simulink library "GenericINSLibrary"  (R2020b)
settings: Solver=VariableStepAuto  StartTime=0.0  StopTime=10.0  RelTol=1e-3
libraries: simulink x44
(part 1 of 6)
settings Model: Creator=Scythe  LastModifiedBy=Scythe
settings DataIOCC: ReturnWorkspaceOutputs=off
settings DebuggingCC: ArithmeticOperatorsInVariantConditions=warning
settings SFSimCC: CustomCodeUndefinedFunction=UseInterfaceOnly

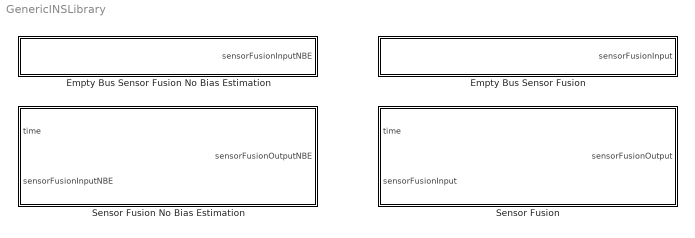
== system GenericINSLibrary ==
  Empty Bus Sensor Fusion : Subsystem
      mask help:
      | Create an empty bus to be used as input for the sensor fusion. By default all measurement values are set to zero and all standard deviations are set to one. A default sensor position is zero and a default sensor orientation equals to an identity matrix.<br><br>
      |
      | Assign values for all fields in the nested initialization bus and assign values for all fields in the nested sensor/IMU bus. All remaining nested sensor busses can optionally be assigned.<br><br>
      |
      | Note that a sensor measurement is only used, if the timestamp of the corresponding sensor increases.
      | Note that the initial state must be given with respect to the position of the IMU.
      mask DialogControl DescGroupVar Prompt: Empty Bus - Sensor Fusion Input
      mask Display: disp('Empty Bus\nSensor Fusion')
  Empty Bus Sensor Fusion No Bias Estimation : Subsystem
      mask help:
      | Create an empty bus to be used as input for the sensor fusion (no bias estimation). By default all measurement values are set to zero and all standard deviations are set to one. A default sensor position is zero and a default sensor orientation equals to an identity matrix.<br><br>
      |
      | Assign values for all fields in the nested initialization bus and assign values for all fields in the nested sensor/IMU bus. All remaining nested sensor busses can optionally be assigned.<br><br>
      |
      | Note that a sensor measurement is only used, if the timestamp of the corresponding sensor increases.
      | Note that the initial state must be given with respect to the position of the IMU.
      mask DialogControl DescGroupVar Prompt: Empty Bus - Sensor Fusion Input (No Bias Estimation)
      mask Display: disp('Empty Bus\nSensor Fusion\n(No Bias Estimation)')
  Sensor Fusion : Subsystem
      mask help:
      | The sensor fusion algorithm that uses multiple sensor data to estimate a motion state and also the inertial sensor biases. An IMU is strictly required to make predictions of the motion. If the IMU is not available for 200 milliseconds, then the filter enters an invalid state and has to be reset/re-initialized. The filter starts in an invalid state and has to be initialized by assigning values to the nested initialization bus and setting the reset flag to true. As long as the reset flag is set to true, the filter is initialized. The sensor fusion output is valid if the filter is initialized and least one prediction using IMU data has been performed.<br><br>
      |
      | <b>INPUT</b><br>
      | <b>time</b><br>
      | The input time source (in seconds) that is used to check for timeout. This time must be monotonically increasing.<br><br>
      |
      | <b>sensorFusionInput</b><br>
      | A bus representing the input to the sensor fusion. An empty input bus can be created by the <i>EmptyBusSensorFusionInput</i> block. Take a look to the mask of this block for more information.<br><br>
      |
      | <b>OUTPUT</b><br>
      | <b>sensorFusionOutput</b><br>
      | A bus representing the output of the sensor fusion. The nested state bus contains the state estimation. The nested info bus contains a valid flag that specifies whether the sensor fusion output is valid or not. Note that the filter gets invalid if IMU measurements timed out.
      mask DialogControl DescGroupVar Prompt: Sensor Fusion
      mask Display: disp('Generic INS\n\nSensor Fusion');
  Sensor Fusion No Bias Estimation : Subsystem
      mask help:
      | The sensor fusion algorithm that uses multiple sensor data to estimate a motion state. An IMU is strictly required to make predictions of the motion. If the IMU is not available for 200 milliseconds, then the filter enters an invalid state and has to be reset/re-initialized. The filter starts in an invalid state and has to be initialized by assigning values to the nested initialization bus and setting the reset flag to true. As long as the reset flag is set to true, the filter is initialized. The sensor fusion output is valid if the filter is initialized and least one prediction using IMU data has been performed.<br><br>
      |
      | <b>INPUT</b><br>
      | <b>time</b><br>
      | The input time source (in seconds) that is used to check for timeout. This time must be monotonically increasing.<br><br>
      |
      | <b>sensorFusionInputNBE</b><br>
      | A bus representing the input to the sensor fusion (no bias estimation). An empty input bus can be created by the <i>EmptyBusSensorFusionInput</i> block. Take a look to the mask of this block for more information.<br><br>
      |
      | <b>OUTPUT</b><br>
      | <b>sensorFusionOutputNBE</b><br>
      | A bus representing the output of the sensor fusion (no bias estimation). The nested state bus contains the state estimation. The nested info bus contains a valid flag that specifies whether the sensor fusion output is valid or not. Note that the filter gets invalid if IMU measurements timed out.
      mask DialogControl DescGroupVar Prompt: Sensor Fusion (No Bias Estimation)
      mask Display: disp('Generic INS\n\nSensor Fusion\n(No Bias Estimation)');

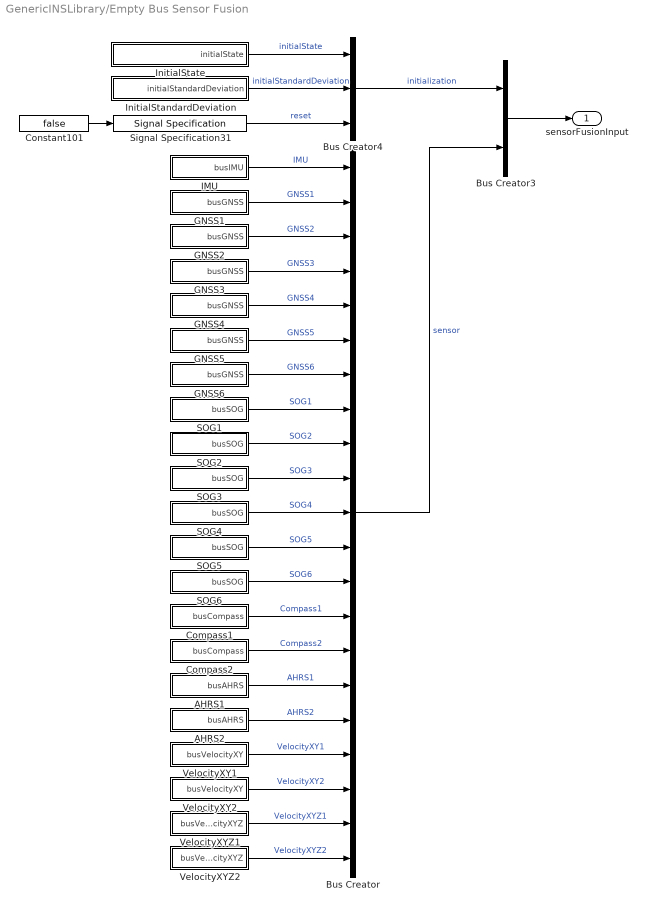
== system GenericINSLibrary/Empty Bus Sensor Fusion ==
  AHRS1 : Subsystem
  AHRS2 : Subsystem
  Bus Creator : BusCreator  Inputs=21
  Bus Creator3 : BusCreator  Inputs=2
  Bus Creator4 : BusCreator  Inputs=3
  Compass1 : Subsystem
  Compass2 : Subsystem
  Constant101 : Constant  Value=false  OutDataTypeStr=boolean
  GNSS1 : Subsystem
  GNSS2 : Subsystem
  GNSS3 : Subsystem
  GNSS4 : Subsystem
  GNSS5 : Subsystem
  GNSS6 : Subsystem
  IMU : Subsystem
  InitialStandardDeviation : Subsystem
  InitialState : Subsystem
  SOG1 : Subsystem
  SOG2 : Subsystem
  SOG3 : Subsystem
  SOG4 : Subsystem
  SOG5 : Subsystem
  SOG6 : Subsystem
  Signal Specification31 : SignalSpecification  OutDataTypeStr=boolean  Dimensions=1
  VelocityXY1 : Subsystem
  VelocityXY2 : Subsystem
  VelocityXYZ1 : Subsystem
  VelocityXYZ2 : Subsystem
  sensorFusionInput : Outport
  wires:
  Bus Creator3/1 -> sensorFusionInput/1
  SOG6/1(busSOG) -> Bus Creator/13  "SOG6"
  AHRS1/1(busAHRS) -> Bus Creator/16  "AHRS1"
  VelocityXY1/1(busVelocityXY) -> Bus Creator/18  "VelocityXY1"
  VelocityXYZ1/1(busVelocityXYZ) -> Bus Creator/20  "VelocityXYZ1"
  SOG5/1(busSOG) -> Bus Creator/12  "SOG5"
  VelocityXY2/1(busVelocityXY) -> Bus Creator/19  "VelocityXY2"
  GNSS4/1(busGNSS) -> Bus Creator/5  "GNSS4"
  GNSS2/1(busGNSS) -> Bus Creator/3  "GNSS2"
  GNSS6/1(busGNSS) -> Bus Creator/7  "GNSS6"
  InitialStandardDeviation/1(initialStandardDeviation) -> Bus Creator4/2  "initialStandardDeviation"
  Bus Creator/1 -> Bus Creator3/2  "sensor"
  SOG1/1(busSOG) -> Bus Creator/8  "SOG1"
  InitialState/1(initialState) -> Bus Creator4/1  "initialState"
  VelocityXYZ2/1(busVelocityXYZ) -> Bus Creator/21  "VelocityXYZ2"
  AHRS2/1(busAHRS) -> Bus Creator/17  "AHRS2"
  Compass2/1(busCompass) -> Bus Creator/15  "Compass2"
  SOG4/1(busSOG) -> Bus Creator/11  "SOG4"
  SOG3/1(busSOG) -> Bus Creator/10  "SOG3"
  Bus Creator4/1 -> Bus Creator3/1  "initialization"
  GNSS5/1(busGNSS) -> Bus Creator/6  "GNSS5"
  Constant101/1 -> Signal Specification31/1
  GNSS3/1(busGNSS) -> Bus Creator/4  "GNSS3"
  Compass1/1(busCompass) -> Bus Creator/14  "Compass1"
  GNSS1/1(busGNSS) -> Bus Creator/2  "GNSS1"
  Signal Specification31/1 -> Bus Creator4/3  "reset"
  IMU/1(busIMU) -> Bus Creator/1  "IMU"
  SOG2/1(busSOG) -> Bus Creator/9  "SOG2"

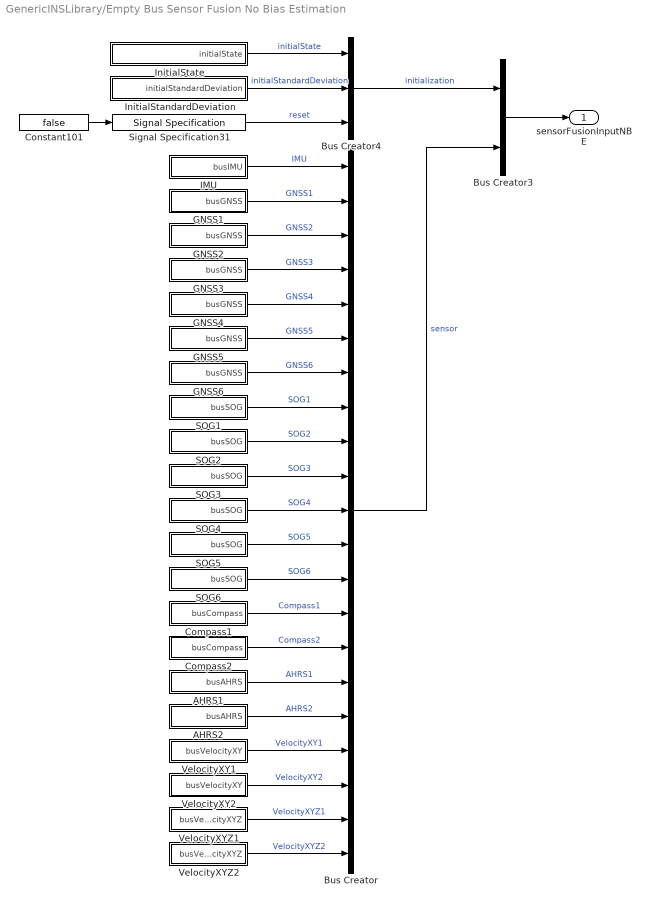
== system GenericINSLibrary/Empty Bus Sensor Fusion No Bias Estimation ==
  AHRS1 : Subsystem
  AHRS2 : Subsystem
  Bus Creator : BusCreator  Inputs=21
  Bus Creator3 : BusCreator  Inputs=2
  Bus Creator4 : BusCreator  Inputs=3
  Compass1 : Subsystem
  Compass2 : Subsystem
  Constant101 : Constant  Value=false  OutDataTypeStr=boolean
  GNSS1 : Subsystem
  GNSS2 : Subsystem
  GNSS3 : Subsystem
  GNSS4 : Subsystem
  GNSS5 : Subsystem
  GNSS6 : Subsystem
  IMU : Subsystem
  InitialStandardDeviation : Subsystem
  InitialState : Subsystem
  SOG1 : Subsystem
  SOG2 : Subsystem
  SOG3 : Subsystem
  SOG4 : Subsystem
  SOG5 : Subsystem
  SOG6 : Subsystem
  Signal Specification31 : SignalSpecification  OutDataTypeStr=boolean  Dimensions=1
  VelocityXY1 : Subsystem
  VelocityXY2 : Subsystem
  VelocityXYZ1 : Subsystem
  VelocityXYZ2 : Subsystem
  sensorFusionInputNBE : Outport
  wires:
  SOG2/1(busSOG) -> Bus Creator/9  "SOG2"
  IMU/1(busIMU) -> Bus Creator/1  "IMU"
  Signal Specification31/1 -> Bus Creator4/3  "reset"
  GNSS1/1(busGNSS) -> Bus Creator/2  "GNSS1"
  Compass1/1(busCompass) -> Bus Creator/14  "Compass1"
  GNSS3/1(busGNSS) -> Bus Creator/4  "GNSS3"
  Constant101/1 -> Signal Specification31/1
  GNSS5/1(busGNSS) -> Bus Creator/6  "GNSS5"
  Bus Creator4/1 -> Bus Creator3/1  "initialization"
  SOG3/1(busSOG) -> Bus Creator/10  "SOG3"
  SOG4/1(busSOG) -> Bus Creator/11  "SOG4"
  Compass2/1(busCompass) -> Bus Creator/15  "Compass2"
  AHRS2/1(busAHRS) -> Bus Creator/17  "AHRS2"
  VelocityXYZ2/1(busVelocityXYZ) -> Bus Creator/21  "VelocityXYZ2"
  InitialState/1(initialState) -> Bus Creator4/1  "initialState"
  SOG1/1(busSOG) -> Bus Creator/8  "SOG1"
  Bus Creator/1 -> Bus Creator3/2  "sensor"
  InitialStandardDeviation/1(initialStandardDeviation) -> Bus Creator4/2  "initialStandardDeviation"
  GNSS6/1(busGNSS) -> Bus Creator/7  "GNSS6"
  GNSS2/1(busGNSS) -> Bus Creator/3  "GNSS2"
  GNSS4/1(busGNSS) -> Bus Creator/5  "GNSS4"
  VelocityXY2/1(busVelocityXY) -> Bus Creator/19  "VelocityXY2"
  SOG5/1(busSOG) -> Bus Creator/12  "SOG5"
  VelocityXYZ1/1(busVelocityXYZ) -> Bus Creator/20  "VelocityXYZ1"
  VelocityXY1/1(busVelocityXY) -> Bus Creator/18  "VelocityXY1"
  AHRS1/1(busAHRS) -> Bus Creator/16  "AHRS1"
  SOG6/1(busSOG) -> Bus Creator/13  "SOG6"
  Bus Creator3/1 -> sensorFusionInputNBE/1

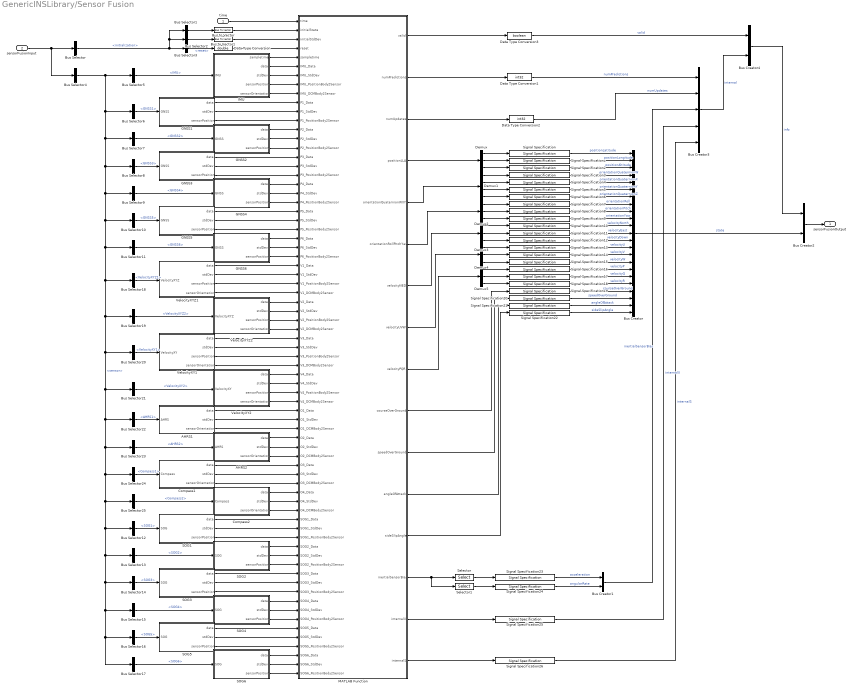
== system GenericINSLibrary/Sensor Fusion ==
  time : Inport  OutDataTypeStr=double  Unit=s  PortDimensions=1
  sensorFusionInput : Inport  Port=2
  AHRS1 : Subsystem
  AHRS2 : Subsystem
  Bus Creator : BusCreator  Inputs=23
  Bus Creator1 : BusCreator  Inputs=2
  Bus Creator2 : BusCreator  Inputs=2
  Bus Creator3 : BusCreator  Inputs=5
  Bus Creator4 : BusCreator  Inputs=2
  Bus Selector : BusSelector  OutputSignals=initialization
  Bus Selector1 : BusSelector  OutputSignals=initialState  OutputAsBus=on
  Bus Selector10 : BusSelector  OutputSignals=GNSS5
  Bus Selector11 : BusSelector  OutputSignals=GNSS6
  Bus Selector12 : BusSelector  OutputSignals=SOG1
  Bus Selector13 : BusSelector  OutputSignals=SOG2
  Bus Selector14 : BusSelector  OutputSignals=SOG3
  Bus Selector15 : BusSelector  OutputSignals=SOG4
  Bus Selector16 : BusSelector  OutputSignals=SOG5
  Bus Selector17 : BusSelector  OutputSignals=SOG6
  Bus Selector18 : BusSelector  OutputSignals=VelocityXYZ1
  Bus Selector19 : BusSelector  OutputSignals=VelocityXYZ2
  Bus Selector2 : BusSelector  OutputSignals=initialStandardDeviation  OutputAsBus=on
  Bus Selector20 : BusSelector  OutputSignals=VelocityXY1
  Bus Selector21 : BusSelector  OutputSignals=VelocityXY2
  Bus Selector22 : BusSelector  OutputSignals=AHRS1
  Bus Selector23 : BusSelector  OutputSignals=AHRS2
  Bus Selector24 : BusSelector  OutputSignals=Compass1
  Bus Selector25 : BusSelector  OutputSignals=Compass2
  Bus Selector3 : BusSelector  OutputSignals=reset
  Bus Selector4 : BusSelector  OutputSignals=sensor
  Bus Selector5 : BusSelector  OutputSignals=IMU
  Bus Selector6 : BusSelector  OutputSignals=GNSS1
  Bus Selector7 : BusSelector  OutputSignals=GNSS2
  Bus Selector8 : BusSelector  OutputSignals=GNSS3
  Bus Selector9 : BusSelector  OutputSignals=GNSS4
  Bus to Vector : BusToVector
  Bus to Vector1 : BusToVector
  Compass1 : Subsystem
  Compass2 : Subsystem
  Data Type Conversion : DataTypeConversion  OutDataTypeStr=double
  Data Type Conversion1 : DataTypeConversion  OutDataTypeStr=int32
  Data Type Conversion2 : DataTypeConversion  OutDataTypeStr=int32
  Data Type Conversion3 : DataTypeConversion  OutDataTypeStr=boolean
  Demux{,2..5} (5 alike) : Demux  Outputs=3
  Demux1 : Demux
  GNSS1 : Subsystem
  GNSS2 : Subsystem
  GNSS3 : Subsystem
  GNSS4 : Subsystem
  GNSS5 : Subsystem
  GNSS6 : Subsystem
  IMU : Subsystem
  MATLAB Function : MATLAB Function  TreatAsAtomicUnit=on
  SOG1 : Subsystem
  SOG2 : Subsystem
  SOG3 : Subsystem
  SOG4 : Subsystem
  SOG5 : Subsystem
  SOG6 : Subsystem
  Selector : Selector  InputPortWidth=6  IndexOptions=Index vector (dialog)  Indices=1:3  OutputSizes=1
  Selector1 : Selector  InputPortWidth=6  IndexOptions=Index vector (dialog)  Indices=4:6  OutputSizes=1
  Signal Specification{,1,7..9,19,21..22} (8 alike) : SignalSpecification  OutDataTypeStr=double  Unit=rad  Dimensions=1
  Signal Specification{10..15,20} (7 alike) : SignalSpecification  OutDataTypeStr=double  Unit=m/s  Dimensions=1
  Signal Specification16 : SignalSpecification  OutDataTypeStr=double  Unit=rad/s  Dimensions=1
  Signal Specification17 : SignalSpecification  OutDataTypeStr=double  Unit=rad/s  Dimensions=1
  Signal Specification18 : SignalSpecification  OutDataTypeStr=double  Unit=rad/s  Dimensions=1
  Signal Specification2 : SignalSpecification  OutDataTypeStr=double  Unit=m  Dimensions=1
  Signal Specification23 : SignalSpecification  OutDataTypeStr=double  Unit=m/s^2  Dimensions=[3 1]
  Signal Specification24 : SignalSpecification  OutDataTypeStr=double  Unit=rad/s  Dimensions=[3 1]
  Signal Specification25 : SignalSpecification  OutDataTypeStr=double  Dimensions=[16 1]
  Signal Specification26 : SignalSpecification  OutDataTypeStr=double  Dimensions=[15 15]
  Signal Specification{3..6} (4 alike) : SignalSpecification  OutDataTypeStr=double  Dimensions=1
  VelocityXY1 : Subsystem
  VelocityXY2 : Subsystem
  VelocityXYZ1 : Subsystem
  VelocityXYZ2 : Subsystem
  sensorFusionOutput : Outport
  wires:
  Bus Selector24/1 -> Compass1/1(Compass)  "<Compass1>"
  Bus Selector7/1 -> GNSS2/1(GNSS)  "<GNSS2>"
  Bus Selector17/1 -> SOG6/1(SOG)  "<SOG6>"
  AHRS1/2(stdDev) -> MATLAB Function/45(O1_StdDev)
  Compass2/3(sensorOrientation) -> MATLAB Function/55(O4_DCMBody2Sensor)
  MATLAB Function/11(speedOverGround) -> Signal Specification20/1
  Selector/1 -> Signal Specification23/1
  AHRS2/2(stdDev) -> MATLAB Function/48(O2_StdDev)
  SOG4/3(sensorPosition) -> MATLAB Function/67(SOG4_PositionBody2Sensor)
  Bus Selector20/1 -> VelocityXY1/1(VelocityXY)  "<VelocityXY1>"
  Demux/3 -> Signal Specification2/1
  Bus Selector16/1 -> SOG5/1(SOG)  "<SOG5>"
  Demux4/2 -> Signal Specification14/1
  SOG3/1(data) -> MATLAB Function/62(SOG3_Data)
  Bus Selector25/1 -> Compass2/1(Compass)  "<Compass2>"
  VelocityXY1/3(sensorPosition) -> MATLAB Function/38(V3_PositionBody2Sensor)
  VelocityXYZ2/2(stdDev) -> MATLAB Function/33(V2_StdDev)
  Signal Specification10/1 -> Bus Creator/11  "velocityNorth"
  GNSS2/1(data) -> MATLAB Function/13(P2_Data)
  Signal Specification3/1 -> Bus Creator/4  "orientationQuaternionW"
  AHRS1/1(data) -> MATLAB Function/44(O1_Data)
  Demux5/2 -> Signal Specification17/1
  SOG4/1(data) -> MATLAB Function/65(SOG4_Data)
  GNSS2/2(stdDev) -> MATLAB Function/14(P2_StdDev)
  Data Type Conversion3/1 -> Bus Creator4/1  "valid"
  MATLAB Function/6(orientationRollPitchYaw) -> Demux2/1
  Demux3/2 -> Signal Specification11/1
  AHRS2/1(data) -> MATLAB Function/47(O2_Data)
  GNSS6/2(stdDev) -> MATLAB Function/26(P6_StdDev)
  Compass1/2(stdDev) -> MATLAB Function/51(O3_StdDev)
  Demux1/2 -> Signal Specification4/1
  Signal Specification22/1 -> Bus Creator/23  "sideSlipAngle"
  Bus Selector1/1 -> Bus to Vector/1
  Bus Selector18/1 -> VelocityXYZ1/1(VelocityXYZ)  "<VelocityXYZ1>"
  MATLAB Function/14(inertialSensorBias) -> Selector/1, Selector1/1
  GNSS6/1(data) -> MATLAB Function/25(P6_Data)
  Signal Specification11/1 -> Bus Creator/12  "velocityEast"
  GNSS1/3(sensorPosition) -> MATLAB Function/12(P1_PositionBody2Sensor)
  Compass1/1(data) -> MATLAB Function/50(O3_Data)
  Compass2/2(stdDev) -> MATLAB Function/54(O4_StdDev)
  Demux1/4 -> Signal Specification6/1
  Demux2/3 -> Signal Specification9/1
  Demux1/3 -> Signal Specification5/1
  Bus Selector13/1 -> SOG2/1(SOG)  "<SOG2>"
  Bus Selector9/1 -> GNSS4/1(GNSS)  "<GNSS4>"
  Data Type Conversion2/1 -> Bus Creator3/2  "numUpdates"
  Bus Creator2/1 -> sensorFusionOutput/1
  Bus to Vector/1 -> MATLAB Function/2(initialState)
  VelocityXYZ1/1(data) -> MATLAB Function/28(V1_Data)
  Signal Specification18/1 -> Bus Creator/19  "velocityR"
  SOG2/3(sensorPosition) -> MATLAB Function/61(SOG2_PositionBody2Sensor)
  SOG6/2(stdDev) -> MATLAB Function/72(SOG6_StdDev)
  SOG3/3(sensorPosition) -> MATLAB Function/64(SOG3_PositionBody2Sensor)
  Signal Specification7/1 -> Bus Creator/8  "orientationRoll"
  Bus to Vector1/1 -> MATLAB Function/3(initialStdDev)
  Bus Creator4/1 -> Bus Creator2/1  "info"
  Signal Specification6/1 -> Bus Creator/7  "orientationQuaternionZ"
  MATLAB Function/4(positionLLA) -> Demux/1
  Bus Selector3/1 -> Data Type Conversion/1  "<reset>"
  GNSS4/3(sensorPosition) -> MATLAB Function/21(P4_PositionBody2Sensor)
  Bus Selector11/1 -> GNSS6/1(GNSS)  "<GNSS6>"
  Signal Specification25/1 -> Bus Creator3/4  "internalX"
  Demux5/1 -> Signal Specification16/1
  Compass2/1(data) -> MATLAB Function/53(O4_Data)
  Bus Creator3/1 -> Bus Creator4/2  "internal"
  Signal Specification17/1 -> Bus Creator/18  "velocityQ"
  time/1 -> MATLAB Function/1(time)
  Demux4/3 -> Signal Specification15/1
  MATLAB Function/13(sideSlipAngle) -> Signal Specification22/1
  MATLAB Function/9(velocityPQR) -> Demux5/1
  Bus Selector/1 -> Bus Selector3/1, Bus Selector1/1, Bus Selector2/1  "<initialization>"
  VelocityXYZ1/2(stdDev) -> MATLAB Function/29(V1_StdDev)
  MATLAB Function/16(internalS) -> Signal Specification26/1
  Demux/1 -> Signal Specification/1
  GNSS5/2(stdDev) -> MATLAB Function/23(P5_StdDev)
  Signal Specification15/1 -> Bus Creator/16  "velocityW"
  SOG5/3(sensorPosition) -> MATLAB Function/70(SOG5_PositionBody2Sensor)
  MATLAB Function/5(orientationQuaternionWXYZ) -> Demux1/1
  GNSS2/3(sensorPosition) -> MATLAB Function/15(P2_PositionBody2Sensor)
  Bus Creator/1 -> Bus Creator2/2  "state"
  MATLAB Function/10(courseOverGround) -> Signal Specification19/1
  VelocityXY1/1(data) -> MATLAB Function/36(V3_Data)
  GNSS4/1(data) -> MATLAB Function/19(P4_Data)
  Demux3/3 -> Signal Specification12/1
  SOG5/1(data) -> MATLAB Function/68(SOG5_Data)
  Signal Specification21/1 -> Bus Creator/22  "angleOfAttack"
  Bus Selector12/1 -> SOG1/1(SOG)  "<SOG1>"
  Demux2/1 -> Signal Specification7/1
  IMU/3(stdDev) -> MATLAB Function/7(IMU_StdDev)
  Demux/2 -> Signal Specification1/1
  SOG2/2(stdDev) -> MATLAB Function/60(SOG2_StdDev)
  Bus Selector8/1 -> GNSS3/1(GNSS)  "<GNSS3>"
  VelocityXY1/4(sensorOrientation) -> MATLAB Function/39(V3_DCMBody2Sensor)
  Signal Specification16/1 -> Bus Creator/17  "velocityP"
  GNSS1/2(stdDev) -> MATLAB Function/11(P1_StdDev)
  SOG1/1(data) -> MATLAB Function/56(SOG1_Data)
  SOG5/2(stdDev) -> MATLAB Function/69(SOG5_StdDev)
  Data Type Conversion1/1 -> Bus Creator3/1  "numPredictions"
  Bus Selector6/1 -> GNSS1/1(GNSS)  "<GNSS1>"
  GNSS6/3(sensorPosition) -> MATLAB Function/27(P6_PositionBody2Sensor)
  sensorFusionInput/1 -> Bus Selector/1, Bus Selector4/1
  MATLAB Function/1(valid) -> Data Type Conversion3/1
  Signal Specification1/1 -> Bus Creator/2  "positionLongitude"
  SOG6/3(sensorPosition) -> MATLAB Function/73(SOG6_PositionBody2Sensor)
  VelocityXY2/3(sensorPosition) -> MATLAB Function/42(V4_PositionBody2Sensor)
  IMU/1(sampletime) -> MATLAB Function/5(sampletime)
  MATLAB Function/15(internalX) -> Signal Specification25/1
  Signal Specification8/1 -> Bus Creator/9  "orientationPitch"
  Bus Selector4/1 -> Bus Selector5/1, Bus Selector6/1, Bus Selector7/1, Bus Selector8/1, Bus Selector9/1, Bus Selector10/1, Bus Selector11/1, Bus Selector18/1, Bus Selector19/1, Bus Selector22/1, Bus Selector12/1, Bus Selector13/1, Bus Selector17/1, Bus Selector16/1, Bus Selector15/1, Bus Selector14/1, Bus Selector25/1, Bus Selector24/1, Bus Selector23/1, Bus Selector21/1, Bus Selector20/1  "<sensor>"
  GNSS4/2(stdDev) -> MATLAB Function/20(P4_StdDev)
  Bus Selector15/1 -> SOG4/1(SOG)  "<SOG4>"
  Demux3/1 -> Signal Specification10/1
  Signal Specification26/1 -> Bus Creator3/5  "internalS"
  Signal Specification9/1 -> Bus Creator/10  "orientationYaw"
  Bus Selector5/1 -> IMU/1(IMU)  "<IMU>"
  Data Type Conversion/1 -> MATLAB Function/4(reset)
  Signal Specification4/1 -> Bus Creator/5  "orientationQuaternionX"
  SOG4/2(stdDev) -> MATLAB Function/66(SOG4_StdDev)
  Bus Selector2/1 -> Bus to Vector1/1
  Compass1/3(sensorOrientation) -> MATLAB Function/52(O3_DCMBody2Sensor)
  GNSS5/3(sensorPosition) -> MATLAB Function/24(P5_PositionBody2Sensor)
  VelocityXY2/4(sensorOrientation) -> MATLAB Function/43(V4_DCMBody2Sensor)
  SOG6/1(data) -> MATLAB Function/71(SOG6_Data)
  Demux5/3 -> Signal Specification18/1
  Bus Selector10/1 -> GNSS5/1(GNSS)  "<GNSS5>"
  Signal Specification12/1 -> Bus Creator/13  "velocityDown"
  VelocityXYZ1/4(sensorOrientation) -> MATLAB Function/31(V1_DCMBody2Sensor)
  IMU/5(sensorOrientation) -> MATLAB Function/9(IMU_DCMBody2Sensor)
  Signal Specification20/1 -> Bus Creator/21  "speedOverGround"
  SOG1/3(sensorPosition) -> MATLAB Function/58(SOG1_PositionBody2Sensor)
  SOG3/2(stdDev) -> MATLAB Function/63(SOG3_StdDev)
  Signal Specification/1 -> Bus Creator/1  "positionLatitude"
  IMU/2(data) -> MATLAB Function/6(IMU_Data)
  Demux4/1 -> Signal Specification13/1
  Signal Specification14/1 -> Bus Creator/15  "velocityV"
  VelocityXY2/2(stdDev) -> MATLAB Function/41(V4_StdDev)
  GNSS1/1(data) -> MATLAB Function/10(P1_Data)
  Bus Creator1/1 -> Bus Creator3/3  "inertialSensorBias"
  GNSS3/3(sensorPosition) -> MATLAB Function/18(P3_PositionBody2Sensor)
  GNSS3/1(data) -> MATLAB Function/16(P3_Data)
  Demux1/1 -> Signal Specification3/1
  VelocityXYZ2/4(sensorOrientation) -> MATLAB Function/35(V2_DCMBody2Sensor)
  VelocityXYZ2/3(sensorPosition) -> MATLAB Function/34(V2_PositionBody2Sensor)
  Signal Specification24/1 -> Bus Creator1/2  "angularRate"
  VelocityXYZ2/1(data) -> MATLAB Function/32(V2_Data)
  MATLAB Function/3(numUpdates) -> Data Type Conversion2/1
  VelocityXY1/2(stdDev) -> MATLAB Function/37(V3_StdDev)
  GNSS3/2(stdDev) -> MATLAB Function/17(P3_StdDev)
  Signal Specification13/1 -> Bus Creator/14  "velocityU"
  Signal Specification19/1 -> Bus Creator/20  "courseOverGround"
  Signal Specification2/1 -> Bus Creator/3  "positionAltitude"
  SOG1/2(stdDev) -> MATLAB Function/57(SOG1_StdDev)
  IMU/4(sensorPosition) -> MATLAB Function/8(IMU_PositionBody2Sensor)
  Bus Selector19/1 -> VelocityXYZ2/1(VelocityXYZ)  "<VelocityXYZ2>"
  MATLAB Function/7(velocityNED) -> Demux3/1
  Bus Selector14/1 -> SOG3/1(SOG)  "<SOG3>"
  VelocityXYZ1/3(sensorPosition) -> MATLAB Function/30(V1_PositionBody2Sensor)
  AHRS1/3(sensorOrientation) -> MATLAB Function/46(O1_DCMBody2Sensor)
  GNSS5/1(data) -> MATLAB Function/22(P5_Data)
  SOG2/1(data) -> MATLAB Function/59(SOG2_Data)
  MATLAB Function/2(numPredictions) -> Data Type Conversion1/1
  AHRS2/3(sensorOrientation) -> MATLAB Function/49(O2_DCMBody2Sensor)
  Selector1/1 -> Signal Specification24/1
  MATLAB Function/8(velocityUVW) -> Demux4/1
  Bus Selector22/1 -> AHRS1/1(AHRS)  "<AHRS1>"
  Demux2/2 -> Signal Specification8/1
  MATLAB Function/12(angleOfAttack) -> Signal Specification21/1
  Signal Specification23/1 -> Bus Creator1/1  "acceleration"
  Bus Selector21/1 -> VelocityXY2/1(VelocityXY)  "<VelocityXY2>"
  Signal Specification5/1 -> Bus Creator/6  "orientationQuaternionY"
  VelocityXY2/1(data) -> MATLAB Function/40(V4_Data)
  Bus Selector23/1 -> AHRS2/1(AHRS)  "<AHRS2>"

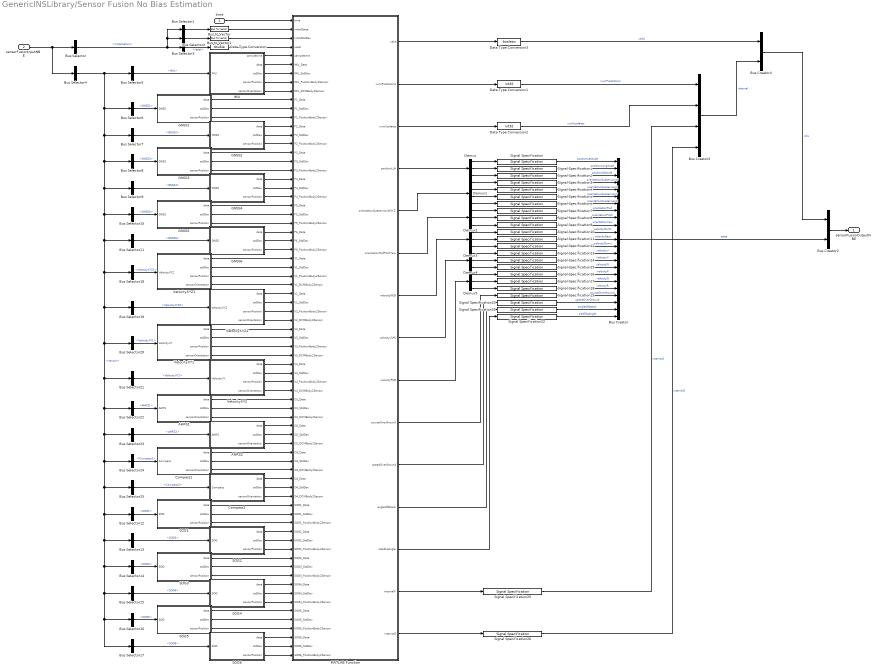
== system GenericINSLibrary/Sensor Fusion No Bias Estimation ==
  time : Inport  OutDataTypeStr=double  Unit=s  PortDimensions=1
  sensorFusionInputNBE : Inport  Port=2
  AHRS1 : Subsystem
  AHRS2 : Subsystem
  Bus Creator : BusCreator  Inputs=23
  Bus Creator2 : BusCreator  Inputs=2
  Bus Creator3 : BusCreator  Inputs=4
  Bus Creator4 : BusCreator  Inputs=2
  Bus Selector : BusSelector  OutputSignals=initialization
  Bus Selector1 : BusSelector  OutputSignals=initialState  OutputAsBus=on
  Bus Selector10 : BusSelector  OutputSignals=GNSS5
  Bus Selector11 : BusSelector  OutputSignals=GNSS6
  Bus Selector12 : BusSelector  OutputSignals=SOG1
  Bus Selector13 : BusSelector  OutputSignals=SOG2
  Bus Selector14 : BusSelector  OutputSignals=SOG3
  Bus Selector15 : BusSelector  OutputSignals=SOG4
  Bus Selector16 : BusSelector  OutputSignals=SOG5
  Bus Selector17 : BusSelector  OutputSignals=SOG6
  Bus Selector18 : BusSelector  OutputSignals=VelocityXYZ1
  Bus Selector19 : BusSelector  OutputSignals=VelocityXYZ2
  Bus Selector2 : BusSelector  OutputSignals=initialStandardDeviation  OutputAsBus=on
  Bus Selector20 : BusSelector  OutputSignals=VelocityXY1
  Bus Selector21 : BusSelector  OutputSignals=VelocityXY2
  Bus Selector22 : BusSelector  OutputSignals=AHRS1
  Bus Selector23 : BusSelector  OutputSignals=AHRS2
  Bus Selector24 : BusSelector  OutputSignals=Compass1
  Bus Selector25 : BusSelector  OutputSignals=Compass2
  Bus Selector3 : BusSelector  OutputSignals=reset
  Bus Selector4 : BusSelector  OutputSignals=sensor
  Bus Selector5 : BusSelector  OutputSignals=IMU
  Bus Selector6 : BusSelector  OutputSignals=GNSS1
  Bus Selector7 : BusSelector  OutputSignals=GNSS2
  Bus Selector8 : BusSelector  OutputSignals=GNSS3
  Bus Selector9 : BusSelector  OutputSignals=GNSS4
  Bus to Vector : BusToVector
  Bus to Vector1 : BusToVector
  Compass1 : Subsystem
  Compass2 : Subsystem
  Data Type Conversion : DataTypeConversion  OutDataTypeStr=double
  Data Type Conversion1 : DataTypeConversion  OutDataTypeStr=int32
  Data Type Conversion2 : DataTypeConversion  OutDataTypeStr=int32
  Data Type Conversion3 : DataTypeConversion  OutDataTypeStr=boolean
  Demux{,2..5} (5 alike) : Demux  Outputs=3
  Demux1 : Demux
  GNSS1 : Subsystem
  GNSS2 : Subsystem
  GNSS3 : Subsystem
  GNSS4 : Subsystem
  GNSS5 : Subsystem
  GNSS6 : Subsystem
  IMU : Subsystem
  MATLAB Function : MATLAB Function  TreatAsAtomicUnit=on
  SOG1 : Subsystem
  SOG2 : Subsystem
  SOG3 : Subsystem
  SOG4 : Subsystem
  SOG5 : Subsystem
  SOG6 : Subsystem
  Signal Specification{,1,7..9,19,21..22} (8 alike) : SignalSpecification  OutDataTypeStr=double  Unit=rad  Dimensions=1
  Signal Specification{10..15,20} (7 alike) : SignalSpecification  OutDataTypeStr=double  Unit=m/s  Dimensions=1
  Signal Specification16 : SignalSpecification  OutDataTypeStr=double  Unit=rad/s  Dimensions=1
  Signal Specification17 : SignalSpecification  OutDataTypeStr=double  Unit=rad/s  Dimensions=1
  Signal Specification18 : SignalSpecification  OutDataTypeStr=double  Unit=rad/s  Dimensions=1
  Signal Specification2 : SignalSpecification  OutDataTypeStr=double  Unit=m  Dimensions=1
  Signal Specification25 : SignalSpecification  OutDataTypeStr=double  Dimensions=[10 1]
  Signal Specification26 : SignalSpecification  OutDataTypeStr=double  Dimensions=[9 9]
  Signal Specification{3..6} (4 alike) : SignalSpecification  OutDataTypeStr=double  Dimensions=1
  VelocityXY1 : Subsystem
  VelocityXY2 : Subsystem
  VelocityXYZ1 : Subsystem
  VelocityXYZ2 : Subsystem
  sensorFusionOutputNBE : Outport
  wires:
  Bus Selector23/1 -> AHRS2/1(AHRS)  "<AHRS2>"
  VelocityXY2/1(data) -> MATLAB Function/40(V4_Data)
  Signal Specification5/1 -> Bus Creator/6  "orientationQuaternionY"
  Bus Selector21/1 -> VelocityXY2/1(VelocityXY)  "<VelocityXY2>"
  MATLAB Function/12(angleOfAttack) -> Signal Specification21/1
  Demux2/2 -> Signal Specification8/1
  Bus Selector22/1 -> AHRS1/1(AHRS)  "<AHRS1>"
  MATLAB Function/8(velocityUVW) -> Demux4/1
  AHRS2/3(sensorOrientation) -> MATLAB Function/49(O2_DCMBody2Sensor)
  MATLAB Function/2(numPredictions) -> Data Type Conversion1/1
  SOG2/1(data) -> MATLAB Function/59(SOG2_Data)
  GNSS5/1(data) -> MATLAB Function/22(P5_Data)
  AHRS1/3(sensorOrientation) -> MATLAB Function/46(O1_DCMBody2Sensor)
  VelocityXYZ1/3(sensorPosition) -> MATLAB Function/30(V1_PositionBody2Sensor)
  Bus Selector14/1 -> SOG3/1(SOG)  "<SOG3>"
  MATLAB Function/7(velocityNED) -> Demux3/1
  Bus Selector19/1 -> VelocityXYZ2/1(VelocityXYZ)  "<VelocityXYZ2>"
  IMU/4(sensorPosition) -> MATLAB Function/8(IMU_PositionBody2Sensor)
  SOG1/2(stdDev) -> MATLAB Function/57(SOG1_StdDev)
  Signal Specification2/1 -> Bus Creator/3  "positionAltitude"
  Signal Specification19/1 -> Bus Creator/20  "courseOverGround"
  Signal Specification13/1 -> Bus Creator/14  "velocityU"
  GNSS3/2(stdDev) -> MATLAB Function/17(P3_StdDev)
  VelocityXY1/2(stdDev) -> MATLAB Function/37(V3_StdDev)
  MATLAB Function/3(numUpdates) -> Data Type Conversion2/1
  VelocityXYZ2/1(data) -> MATLAB Function/32(V2_Data)
  VelocityXYZ2/3(sensorPosition) -> MATLAB Function/34(V2_PositionBody2Sensor)
  VelocityXYZ2/4(sensorOrientation) -> MATLAB Function/35(V2_DCMBody2Sensor)
  Demux1/1 -> Signal Specification3/1
  GNSS3/1(data) -> MATLAB Function/16(P3_Data)
  GNSS3/3(sensorPosition) -> MATLAB Function/18(P3_PositionBody2Sensor)
  GNSS1/1(data) -> MATLAB Function/10(P1_Data)
  VelocityXY2/2(stdDev) -> MATLAB Function/41(V4_StdDev)
  Signal Specification14/1 -> Bus Creator/15  "velocityV"
  Demux4/1 -> Signal Specification13/1
  IMU/2(data) -> MATLAB Function/6(IMU_Data)
  Signal Specification/1 -> Bus Creator/1  "positionLatitude"
  SOG3/2(stdDev) -> MATLAB Function/63(SOG3_StdDev)
  SOG1/3(sensorPosition) -> MATLAB Function/58(SOG1_PositionBody2Sensor)
  Signal Specification20/1 -> Bus Creator/21  "speedOverGround"
  IMU/5(sensorOrientation) -> MATLAB Function/9(IMU_DCMBody2Sensor)
  VelocityXYZ1/4(sensorOrientation) -> MATLAB Function/31(V1_DCMBody2Sensor)
  Signal Specification12/1 -> Bus Creator/13  "velocityDown"
  Bus Selector10/1 -> GNSS5/1(GNSS)  "<GNSS5>"
  Demux5/3 -> Signal Specification18/1
  SOG6/1(data) -> MATLAB Function/71(SOG6_Data)
  VelocityXY2/4(sensorOrientation) -> MATLAB Function/43(V4_DCMBody2Sensor)
  GNSS5/3(sensorPosition) -> MATLAB Function/24(P5_PositionBody2Sensor)
  Compass1/3(sensorOrientation) -> MATLAB Function/52(O3_DCMBody2Sensor)
  Bus Selector2/1 -> Bus to Vector1/1
  SOG4/2(stdDev) -> MATLAB Function/66(SOG4_StdDev)
  Signal Specification4/1 -> Bus Creator/5  "orientationQuaternionX"
  Data Type Conversion/1 -> MATLAB Function/4(reset)
  Bus Selector5/1 -> IMU/1(IMU)  "<IMU>"
  Signal Specification9/1 -> Bus Creator/10  "orientationYaw"
  Signal Specification26/1 -> Bus Creator3/4  "internalS"
  Demux3/1 -> Signal Specification10/1
  Bus Selector15/1 -> SOG4/1(SOG)  "<SOG4>"
  GNSS4/2(stdDev) -> MATLAB Function/20(P4_StdDev)
  Bus Selector4/1 -> Bus Selector20/1, Bus Selector21/1, Bus Selector23/1, Bus Selector24/1, Bus Selector25/1, Bus Selector14/1, Bus Selector15/1, Bus Selector16/1, Bus Selector17/1, Bus Selector13/1, Bus Selector12/1, Bus Selector22/1, Bus Selector19/1, Bus Selector18/1, Bus Selector11/1, Bus Selector10/1, Bus Selector9/1, Bus Selector8/1, Bus Selector7/1, Bus Selector6/1, Bus Selector5/1  "<sensor>"
  Signal Specification8/1 -> Bus Creator/9  "orientationPitch"
  MATLAB Function/14(internalX) -> Signal Specification25/1
  IMU/1(sampletime) -> MATLAB Function/5(sampletime)
  VelocityXY2/3(sensorPosition) -> MATLAB Function/42(V4_PositionBody2Sensor)
  SOG6/3(sensorPosition) -> MATLAB Function/73(SOG6_PositionBody2Sensor)
  Signal Specification1/1 -> Bus Creator/2  "positionLongitude"
  MATLAB Function/1(valid) -> Data Type Conversion3/1
  sensorFusionInputNBE/1 -> Bus Selector4/1, Bus Selector/1
  GNSS6/3(sensorPosition) -> MATLAB Function/27(P6_PositionBody2Sensor)
  Bus Selector6/1 -> GNSS1/1(GNSS)  "<GNSS1>"
  Data Type Conversion1/1 -> Bus Creator3/1  "numPredictions"
  SOG5/2(stdDev) -> MATLAB Function/69(SOG5_StdDev)
  SOG1/1(data) -> MATLAB Function/56(SOG1_Data)
  GNSS1/2(stdDev) -> MATLAB Function/11(P1_StdDev)
  Signal Specification16/1 -> Bus Creator/17  "velocityP"
  VelocityXY1/4(sensorOrientation) -> MATLAB Function/39(V3_DCMBody2Sensor)
  Bus Selector8/1 -> GNSS3/1(GNSS)  "<GNSS3>"
  SOG2/2(stdDev) -> MATLAB Function/60(SOG2_StdDev)
  Demux/2 -> Signal Specification1/1
  IMU/3(stdDev) -> MATLAB Function/7(IMU_StdDev)
  Demux2/1 -> Signal Specification7/1
  Bus Selector12/1 -> SOG1/1(SOG)  "<SOG1>"
  Signal Specification21/1 -> Bus Creator/22  "angleOfAttack"
  SOG5/1(data) -> MATLAB Function/68(SOG5_Data)
  Demux3/3 -> Signal Specification12/1
  GNSS4/1(data) -> MATLAB Function/19(P4_Data)
  VelocityXY1/1(data) -> MATLAB Function/36(V3_Data)
  MATLAB Function/10(courseOverGround) -> Signal Specification19/1
  Bus Creator/1 -> Bus Creator2/2  "state"
  GNSS2/3(sensorPosition) -> MATLAB Function/15(P2_PositionBody2Sensor)
  MATLAB Function/5(orientationQuaternionWXYZ) -> Demux1/1
  SOG5/3(sensorPosition) -> MATLAB Function/70(SOG5_PositionBody2Sensor)
  Signal Specification15/1 -> Bus Creator/16  "velocityW"
  GNSS5/2(stdDev) -> MATLAB Function/23(P5_StdDev)
  Demux/1 -> Signal Specification/1
  MATLAB Function/15(internalS) -> Signal Specification26/1
  VelocityXYZ1/2(stdDev) -> MATLAB Function/29(V1_StdDev)
  Bus Selector/1 -> Bus Selector2/1, Bus Selector1/1, Bus Selector3/1  "<initialization>"
  MATLAB Function/9(velocityPQR) -> Demux5/1
  MATLAB Function/13(sideSlipAngle) -> Signal Specification22/1
  Demux4/3 -> Signal Specification15/1
  time/1 -> MATLAB Function/1(time)
  Signal Specification17/1 -> Bus Creator/18  "velocityQ"
  Bus Creator3/1 -> Bus Creator4/2  "internal"
  Compass2/1(data) -> MATLAB Function/53(O4_Data)
  Demux5/1 -> Signal Specification16/1
  Signal Specification25/1 -> Bus Creator3/3  "internalX"
  Bus Selector11/1 -> GNSS6/1(GNSS)  "<GNSS6>"
  GNSS4/3(sensorPosition) -> MATLAB Function/21(P4_PositionBody2Sensor)
  Bus Selector3/1 -> Data Type Conversion/1  "<reset>"
  MATLAB Function/4(positionLLA) -> Demux/1
  Signal Specification6/1 -> Bus Creator/7  "orientationQuaternionZ"
  Bus Creator4/1 -> Bus Creator2/1  "info"
  Bus to Vector1/1 -> MATLAB Function/3(initialStdDev)
  Signal Specification7/1 -> Bus Creator/8  "orientationRoll"
  SOG3/3(sensorPosition) -> MATLAB Function/64(SOG3_PositionBody2Sensor)
  SOG6/2(stdDev) -> MATLAB Function/72(SOG6_StdDev)
  SOG2/3(sensorPosition) -> MATLAB Function/61(SOG2_PositionBody2Sensor)
  Signal Specification18/1 -> Bus Creator/19  "velocityR"
  VelocityXYZ1/1(data) -> MATLAB Function/28(V1_Data)
  Bus to Vector/1 -> MATLAB Function/2(initialState)
  Bus Creator2/1 -> sensorFusionOutputNBE/1
  Data Type Conversion2/1 -> Bus Creator3/2  "numUpdates"
  Bus Selector9/1 -> GNSS4/1(GNSS)  "<GNSS4>"
  Bus Selector13/1 -> SOG2/1(SOG)  "<SOG2>"
  Demux1/3 -> Signal Specification5/1
  Demux2/3 -> Signal Specification9/1
  Demux1/4 -> Signal Specification6/1
  Compass2/2(stdDev) -> MATLAB Function/54(O4_StdDev)
  Compass1/1(data) -> MATLAB Function/50(O3_Data)
  GNSS1/3(sensorPosition) -> MATLAB Function/12(P1_PositionBody2Sensor)
  Signal Specification11/1 -> Bus Creator/12  "velocityEast"
  GNSS6/1(data) -> MATLAB Function/25(P6_Data)
  Bus Selector18/1 -> VelocityXYZ1/1(VelocityXYZ)  "<VelocityXYZ1>"
  Bus Selector1/1 -> Bus to Vector/1
  Signal Specification22/1 -> Bus Creator/23  "sideSlipAngle"
  Demux1/2 -> Signal Specification4/1
  Compass1/2(stdDev) -> MATLAB Function/51(O3_StdDev)
  GNSS6/2(stdDev) -> MATLAB Function/26(P6_StdDev)
  AHRS2/1(data) -> MATLAB Function/47(O2_Data)
  Demux3/2 -> Signal Specification11/1
  MATLAB Function/6(orientationRollPitchYaw) -> Demux2/1
  Data Type Conversion3/1 -> Bus Creator4/1  "valid"
  GNSS2/2(stdDev) -> MATLAB Function/14(P2_StdDev)
  SOG4/1(data) -> MATLAB Function/65(SOG4_Data)
  Demux5/2 -> Signal Specification17/1
  AHRS1/1(data) -> MATLAB Function/44(O1_Data)
  Signal Specification3/1 -> Bus Creator/4  "orientationQuaternionW"
  GNSS2/1(data) -> MATLAB Function/13(P2_Data)
  Signal Specification10/1 -> Bus Creator/11  "velocityNorth"
  VelocityXYZ2/2(stdDev) -> MATLAB Function/33(V2_StdDev)
  VelocityXY1/3(sensorPosition) -> MATLAB Function/38(V3_PositionBody2Sensor)
  Bus Selector25/1 -> Compass2/1(Compass)  "<Compass2>"
  SOG3/1(data) -> MATLAB Function/62(SOG3_Data)
  Demux4/2 -> Signal Specification14/1
  Bus Selector16/1 -> SOG5/1(SOG)  "<SOG5>"
  Demux/3 -> Signal Specification2/1
  Bus Selector20/1 -> VelocityXY1/1(VelocityXY)  "<VelocityXY1>"
  SOG4/3(sensorPosition) -> MATLAB Function/67(SOG4_PositionBody2Sensor)
  AHRS2/2(stdDev) -> MATLAB Function/48(O2_StdDev)
  MATLAB Function/11(speedOverGround) -> Signal Specification20/1
  Compass2/3(sensorOrientation) -> MATLAB Function/55(O4_DCMBody2Sensor)
  AHRS1/2(stdDev) -> MATLAB Function/45(O1_StdDev)
  Bus Selector17/1 -> SOG6/1(SOG)  "<SOG6>"
  Bus Selector7/1 -> GNSS2/1(GNSS)  "<GNSS2>"
  Bus Selector24/1 -> Compass1/1(Compass)  "<Compass1>"

== system GenericINSLibrary/Empty Bus Sensor Fusion/AHRS1 ==
  Bus Creator : BusCreator  Inputs=1
  Bus Creator1 : BusCreator  Inputs=3
  Bus Creator2 : BusCreator  Inputs=3
  Bus Creator3 : BusCreator  Inputs=4
  Constant1 : Constant  OutDataTypeStr=double
  Constant2 : Constant  OutDataTypeStr=double
  Constant{3..4,75..76} (4 alike) : Constant  Value=0  OutDataTypeStr=double
  Constant71 : Constant  Value=eye(3)  OutDataTypeStr=double
  Constant72 : Constant  OutDataTypeStr=double
  Signal Specification : SignalSpecification  OutDataTypeStr=double  Dimensions=[3 3]
  Signal Specification{1..3,5..7} (6 alike) : SignalSpecification  OutDataTypeStr=double  Unit=rad  Dimensions=1
  Signal Specification4 : SignalSpecification  OutDataTypeStr=double  Unit=s  Dimensions=1
  busAHRS : Outport
  wires:
  Constant4/1 -> Signal Specification7/1
  Constant3/1 -> Signal Specification6/1
  Signal Specification7/1 -> Bus Creator3/4  "yaw"
  Signal Specification6/1 -> Bus Creator3/3  "pitch"
  Signal Specification5/1 -> Bus Creator2/3  "yaw"
  Signal Specification3/1 -> Bus Creator2/2  "pitch"
  Constant2/1 -> Signal Specification5/1
  Constant1/1 -> Signal Specification3/1
  Signal Specification2/1 -> Bus Creator3/2  "roll"
  Constant72/1 -> Signal Specification1/1
  Signal Specification1/1 -> Bus Creator2/1  "roll"
  Constant76/1 -> Signal Specification2/1
  Constant71/1 -> Signal Specification/1
  Bus Creator2/1 -> Bus Creator1/2  "standardDeviation"
  Bus Creator3/1 -> Bus Creator1/3  "measurement"
  Bus Creator/1 -> Bus Creator1/1  "alignment"
  Signal Specification/1 -> Bus Creator/1  "rotationMatrixBodyToSensor"
  Constant75/1 -> Signal Specification4/1
  Signal Specification4/1 -> Bus Creator3/1  "timestamp"
  Bus Creator1/1 -> busAHRS/1

== system GenericINSLibrary/Empty Bus Sensor Fusion/AHRS2 ==
  Bus Creator : BusCreator  Inputs=1
  Bus Creator1 : BusCreator  Inputs=3
  Bus Creator2 : BusCreator  Inputs=3
  Bus Creator3 : BusCreator  Inputs=4
  Constant1 : Constant  OutDataTypeStr=double
  Constant2 : Constant  OutDataTypeStr=double
  Constant{3..4,75..76} (4 alike) : Constant  Value=0  OutDataTypeStr=double
  Constant71 : Constant  Value=eye(3)  OutDataTypeStr=double
  Constant72 : Constant  OutDataTypeStr=double
  Signal Specification : SignalSpecification  OutDataTypeStr=double  Dimensions=[3 3]
  Signal Specification{1..3,5..7} (6 alike) : SignalSpecification  OutDataTypeStr=double  Unit=rad  Dimensions=1
  Signal Specification4 : SignalSpecification  OutDataTypeStr=double  Unit=s  Dimensions=1
  busAHRS : Outport
  wires:
  Bus Creator1/1 -> busAHRS/1
  Signal Specification4/1 -> Bus Creator3/1  "timestamp"
  Constant75/1 -> Signal Specification4/1
  Signal Specification/1 -> Bus Creator/1  "rotationMatrixBodyToSensor"
  Bus Creator/1 -> Bus Creator1/1  "alignment"
  Bus Creator3/1 -> Bus Creator1/3  "measurement"
  Bus Creator2/1 -> Bus Creator1/2  "standardDeviation"
  Constant71/1 -> Signal Specification/1
  Constant76/1 -> Signal Specification2/1
  Signal Specification1/1 -> Bus Creator2/1  "roll"
  Constant72/1 -> Signal Specification1/1
  Signal Specification2/1 -> Bus Creator3/2  "roll"
  Constant1/1 -> Signal Specification3/1
  Constant2/1 -> Signal Specification5/1
  Signal Specification3/1 -> Bus Creator2/2  "pitch"
  Signal Specification5/1 -> Bus Creator2/3  "yaw"
  Signal Specification6/1 -> Bus Creator3/3  "pitch"
  Signal Specification7/1 -> Bus Creator3/4  "yaw"
  Constant3/1 -> Signal Specification6/1
  Constant4/1 -> Signal Specification7/1

== system GenericINSLibrary/Empty Bus Sensor Fusion/Compass1 ==
  Bus Creator : BusCreator  Inputs=1
  Bus Creator1 : BusCreator  Inputs=3
  Bus Creator2 : BusCreator  Inputs=1
  Bus Creator3 : BusCreator  Inputs=2
  Constant71 : Constant  Value=eye(3)  OutDataTypeStr=double
  Constant72 : Constant  OutDataTypeStr=double
  Constant75 : Constant  Value=0  OutDataTypeStr=double
  Constant76 : Constant  Value=0  OutDataTypeStr=double
  Signal Specification : SignalSpecification  OutDataTypeStr=double  Dimensions=[3 3]
  Signal Specification1 : SignalSpecification  OutDataTypeStr=double  Unit=rad  Dimensions=1
  Signal Specification2 : SignalSpecification  OutDataTypeStr=double  Unit=rad  Dimensions=1
  Signal Specification4 : SignalSpecification  OutDataTypeStr=double  Unit=s  Dimensions=1
  busCompass : Outport
  wires:
  Signal Specification2/1 -> Bus Creator3/2  "yaw"
  Constant72/1 -> Signal Specification1/1
  Signal Specification1/1 -> Bus Creator2/1  "yaw"
  Constant76/1 -> Signal Specification2/1
  Constant71/1 -> Signal Specification/1
  Bus Creator2/1 -> Bus Creator1/2  "standardDeviation"
  Bus Creator3/1 -> Bus Creator1/3  "measurement"
  Bus Creator/1 -> Bus Creator1/1  "alignment"
  Signal Specification/1 -> Bus Creator/1  "rotationMatrixBodyToSensor"
  Constant75/1 -> Signal Specification4/1
  Signal Specification4/1 -> Bus Creator3/1  "timestamp"
  Bus Creator1/1 -> busCompass/1

== system GenericINSLibrary/Empty Bus Sensor Fusion/Compass2 ==
  Bus Creator : BusCreator  Inputs=1
  Bus Creator1 : BusCreator  Inputs=3
  Bus Creator2 : BusCreator  Inputs=1
  Bus Creator3 : BusCreator  Inputs=2
  Constant71 : Constant  Value=eye(3)  OutDataTypeStr=double
  Constant72 : Constant  OutDataTypeStr=double
  Constant75 : Constant  Value=0  OutDataTypeStr=double
  Constant76 : Constant  Value=0  OutDataTypeStr=double
  Signal Specification : SignalSpecification  OutDataTypeStr=double  Dimensions=[3 3]
  Signal Specification1 : SignalSpecification  OutDataTypeStr=double  Unit=rad  Dimensions=1
  Signal Specification2 : SignalSpecification  OutDataTypeStr=double  Unit=rad  Dimensions=1
  Signal Specification4 : SignalSpecification  OutDataTypeStr=double  Unit=s  Dimensions=1
  busCompass : Outport
  wires:
  Bus Creator1/1 -> busCompass/1
  Signal Specification4/1 -> Bus Creator3/1  "timestamp"
  Constant75/1 -> Signal Specification4/1
  Signal Specification/1 -> Bus Creator/1  "rotationMatrixBodyToSensor"
  Bus Creator/1 -> Bus Creator1/1  "alignment"
  Bus Creator3/1 -> Bus Creator1/3  "measurement"
  Bus Creator2/1 -> Bus Creator1/2  "standardDeviation"
  Constant71/1 -> Signal Specification/1
  Constant76/1 -> Signal Specification2/1
  Signal Specification1/1 -> Bus Creator2/1  "yaw"
  Constant72/1 -> Signal Specification1/1
  Signal Specification2/1 -> Bus Creator3/2  "yaw"

== system GenericINSLibrary/Empty Bus Sensor Fusion/GNSS1 ==
  Bus Creator : BusCreator  Inputs=1
  Bus Creator1 : BusCreator  Inputs=3
  Bus Creator2 : BusCreator  Inputs=3
  Bus Creator3 : BusCreator  Inputs=4
  Constant71 : Constant  Value=[0;0;0]  OutDataTypeStr=double
  Constant72 : Constant  OutDataTypeStr=double
  Constant73 : Constant  OutDataTypeStr=double
  Constant74 : Constant  OutDataTypeStr=double
  Constant{75..78} (4 alike) : Constant  Value=0  OutDataTypeStr=double
  Signal Specification : SignalSpecification  OutDataTypeStr=double  Unit=m  Dimensions=3
  Signal Specification{1..3,7} (4 alike) : SignalSpecification  OutDataTypeStr=double  Unit=m  Dimensions=1
  Signal Specification4 : SignalSpecification  OutDataTypeStr=double  Unit=s  Dimensions=1
  Signal Specification5 : SignalSpecification  OutDataTypeStr=double  Unit=rad  Dimensions=1
  Signal Specification6 : SignalSpecification  OutDataTypeStr=double  Unit=rad  Dimensions=1
  busGNSS : Outport
  wires:
  Bus Creator1/1 -> busGNSS/1
  Signal Specification4/1 -> Bus Creator3/1  "timestamp"
  Constant75/1 -> Signal Specification4/1
  Signal Specification/1 -> Bus Creator/1  "positionBodyToSensor"
  Signal Specification2/1 -> Bus Creator2/2  "east"
  Constant74/1 -> Signal Specification3/1
  Bus Creator/1 -> Bus Creator1/1  "alignment"
  Signal Specification3/1 -> Bus Creator2/3  "down"
  Bus Creator3/1 -> Bus Creator1/3  "measurement"
  Bus Creator2/1 -> Bus Creator1/2  "standardDeviation"
  Signal Specification5/1 -> Bus Creator3/2  "latitude"
  Constant78/1 -> Signal Specification7/1
  Signal Specification7/1 -> Bus Creator3/4  "altitude"
  Constant73/1 -> Signal Specification2/1
  Constant71/1 -> Signal Specification/1
  Constant76/1 -> Signal Specification5/1
  Constant77/1 -> Signal Specification6/1
  Signal Specification1/1 -> Bus Creator2/1  "north"
  Constant72/1 -> Signal Specification1/1
  Signal Specification6/1 -> Bus Creator3/3  "longitude"

== system GenericINSLibrary/Empty Bus Sensor Fusion/GNSS2 ==
  Bus Creator : BusCreator  Inputs=1
  Bus Creator1 : BusCreator  Inputs=3
  Bus Creator2 : BusCreator  Inputs=3
  Bus Creator3 : BusCreator  Inputs=4
  Constant71 : Constant  Value=[0;0;0]  OutDataTypeStr=double
  Constant72 : Constant  OutDataTypeStr=double
  Constant73 : Constant  OutDataTypeStr=double
  Constant74 : Constant  OutDataTypeStr=double
  Constant{75..78} (4 alike) : Constant  Value=0  OutDataTypeStr=double
  Signal Specification : SignalSpecification  OutDataTypeStr=double  Unit=m  Dimensions=3
  Signal Specification{1..3,7} (4 alike) : SignalSpecification  OutDataTypeStr=double  Unit=m  Dimensions=1
  Signal Specification4 : SignalSpecification  OutDataTypeStr=double  Unit=s  Dimensions=1
  Signal Specification5 : SignalSpecification  OutDataTypeStr=double  Unit=rad  Dimensions=1
  Signal Specification6 : SignalSpecification  OutDataTypeStr=double  Unit=rad  Dimensions=1
  busGNSS : Outport
  wires:
  Signal Specification6/1 -> Bus Creator3/3  "longitude"
  Constant72/1 -> Signal Specification1/1
  Signal Specification1/1 -> Bus Creator2/1  "north"
  Constant77/1 -> Signal Specification6/1
  Constant76/1 -> Signal Specification5/1
  Constant71/1 -> Signal Specification/1
  Constant73/1 -> Signal Specification2/1
  Signal Specification7/1 -> Bus Creator3/4  "altitude"
  Constant78/1 -> Signal Specification7/1
  Signal Specification5/1 -> Bus Creator3/2  "latitude"
  Bus Creator2/1 -> Bus Creator1/2  "standardDeviation"
  Bus Creator3/1 -> Bus Creator1/3  "measurement"
  Signal Specification3/1 -> Bus Creator2/3  "down"
  Bus Creator/1 -> Bus Creator1/1  "alignment"
  Constant74/1 -> Signal Specification3/1
  Signal Specification2/1 -> Bus Creator2/2  "east"
  Signal Specification/1 -> Bus Creator/1  "positionBodyToSensor"
  Constant75/1 -> Signal Specification4/1
  Signal Specification4/1 -> Bus Creator3/1  "timestamp"
  Bus Creator1/1 -> busGNSS/1

== system GenericINSLibrary/Empty Bus Sensor Fusion/GNSS3 ==
  Bus Creator : BusCreator  Inputs=1
  Bus Creator1 : BusCreator  Inputs=3
  Bus Creator2 : BusCreator  Inputs=3
  Bus Creator3 : BusCreator  Inputs=4
  Constant71 : Constant  Value=[0;0;0]  OutDataTypeStr=double
  Constant72 : Constant  OutDataTypeStr=double
  Constant73 : Constant  OutDataTypeStr=double
  Constant74 : Constant  OutDataTypeStr=double
  Constant{75..78} (4 alike) : Constant  Value=0  OutDataTypeStr=double
  Signal Specification : SignalSpecification  OutDataTypeStr=double  Unit=m  Dimensions=3
  Signal Specification{1..3,7} (4 alike) : SignalSpecification  OutDataTypeStr=double  Unit=m  Dimensions=1
  Signal Specification4 : SignalSpecification  OutDataTypeStr=double  Unit=s  Dimensions=1
  Signal Specification5 : SignalSpecification  OutDataTypeStr=double  Unit=rad  Dimensions=1
  Signal Specification6 : SignalSpecification  OutDataTypeStr=double  Unit=rad  Dimensions=1
  busGNSS : Outport
  wires:
  Bus Creator1/1 -> busGNSS/1
  Signal Specification4/1 -> Bus Creator3/1  "timestamp"
  Constant75/1 -> Signal Specification4/1
  Signal Specification/1 -> Bus Creator/1  "positionBodyToSensor"
  Signal Specification2/1 -> Bus Creator2/2  "east"
  Constant74/1 -> Signal Specification3/1
  Bus Creator/1 -> Bus Creator1/1  "alignment"
  Signal Specification3/1 -> Bus Creator2/3  "down"
  Bus Creator3/1 -> Bus Creator1/3  "measurement"
  Bus Creator2/1 -> Bus Creator1/2  "standardDeviation"
  Signal Specification5/1 -> Bus Creator3/2  "latitude"
  Constant78/1 -> Signal Specification7/1
  Signal Specification7/1 -> Bus Creator3/4  "altitude"
  Constant73/1 -> Signal Specification2/1
  Constant71/1 -> Signal Specification/1
  Constant76/1 -> Signal Specification5/1
  Constant77/1 -> Signal Specification6/1
  Signal Specification1/1 -> Bus Creator2/1  "north"
  Constant72/1 -> Signal Specification1/1
  Signal Specification6/1 -> Bus Creator3/3  "longitude"
